simulink model "neural_network_and_real_data"  (Simulink 5.0)
settings: Solver=ode45  StartTime=0.0  StopTime=96  RelTol=1e-3
libraries: neural x7
settings Model: LastModifiedBy=Admin

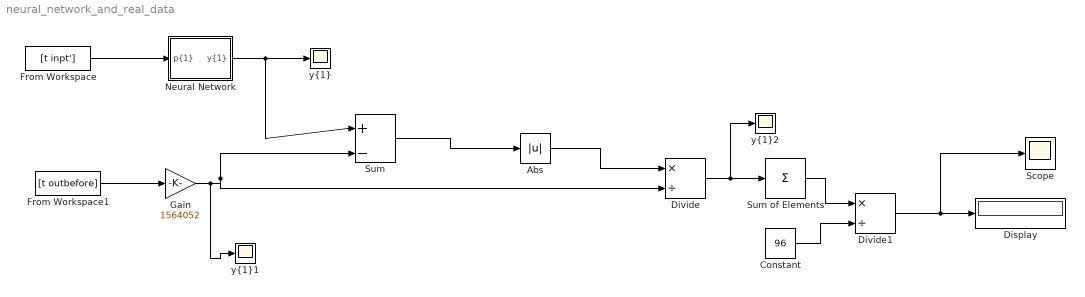
== system neural_network_and_real_data ==
  Abs : Abs  SaturateOnIntegerOverflow=on
  Constant : Constant  Value=96
  Display : Display
  Divide : Product  Inputs=*/  ShowAdditionalParam=on  OutDataTypeMode=double  OutScaling=2^-10
  Divide1 : Product  Inputs=*/  ShowAdditionalParam=on  OutDataTypeMode=double  OutScaling=2^-10
  From Workspace : FromWorkspace  VariableName=[t inpt']  SampleTime=0
  From Workspace1 : FromWorkspace  VariableName=[t outbefore]  SampleTime=0
  Gain : Gain  Gain=1564052  SaturateOnIntegerOverflow=on
  Neural Network : Subsystem
  Scope : Scope
  Sum : Sum  Inputs=|+-  SaturateOnIntegerOverflow=on
  Sum of Elements : Sum  Inputs=+  ShowAdditionalParam=on  OutDataTypeMode=double  OutScaling=2^-10
  "y{1}" : Scope
      settings: DataFormat=Array
  "y{1}1" : Scope
      settings: SaveName=ScopeData2  DataFormat=Array
  "y{1}2" : Scope
      settings: SaveName=ScopeData3  DataFormat=Array
  wires:
  From Workspace1/1 -> Gain/1
  Sum/1 -> Abs/1
  Abs/1 -> Divide/1
  Gain/1 -> Sum/2, Divide/2, "y{1}1"/1
  Divide/1 -> Sum of Elements/1, "y{1}2"/1
  Sum of Elements/1 -> Divide1/1
  Divide1/1 -> Display/1, Scope/1
  Constant/1 -> Divide1/2
  From Workspace/1 -> Neural Network/1("p{1}")
  Neural Network/1("y{1}") -> "y{1}"/1, Sum/1

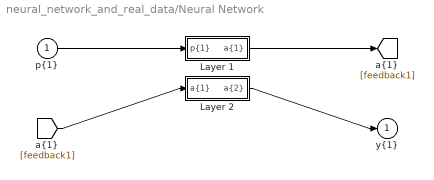
== system neural_network_and_real_data/Neural Network ==
  "p{1}" : Inport  PortDimensions=14  SampleTime=1
  Layer 1 : Subsystem
  Layer 2 : Subsystem
  "y{1}" : Outport  InitialOutput=0
  wires:
  "p{1}"/1 -> Layer 1/1("p{1}")
  Layer 1/1("a{1}") -> [feedback1]
  [feedback1] -> Layer 2/1("a{1} ")
  Layer 2/1("a{2}") -> "y{1}"/1

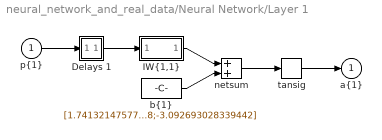
== system neural_network_and_real_data/Neural Network/Layer 1 ==
  "p{1}" : Inport  PortDimensions=14  SampleTime=1
  Delays 1 : Subsystem
      mask Display: disp('TDL')
  "IW{1,1}" : Subsystem
      mask Display: disp('weight')
  "b{1}" : Constant  Value=[1.7413214757740016;0.69735815383961486;-8.2527879365355368;-3.092693028339442]
      mask Display: disp('bias')
  netsum : Sum  Inputs=2  SaturateOnIntegerOverflow=on  InputSameDT=on
  tansig : neural/Transfer Functions/tansig
  "a{1}" : Outport  InitialOutput=[0;0;0;0]
  wires:
  "p{1}"/1 -> Delays 1/1("p{1}")
  Delays 1/1("pd{1,1}") -> "IW{1,1}"/1("pd{1,1}")
  "IW{1,1}"/1("iz{1,1}") -> netsum/1
  "b{1}"/1 -> netsum/2
  netsum/1 -> tansig/1
  tansig/1 -> "a{1}"/1

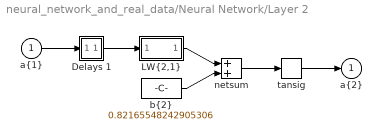
== system neural_network_and_real_data/Neural Network/Layer 2 ==
  "a{1} " : Inport  PortDimensions=4  SampleTime=1
  Delays 1 : Subsystem
      mask Display: disp('TDL')
  "LW{2,1}" : Subsystem
      mask Display: disp('weight')
  "b{2}" : Constant  Value=0.82165548242905306
      mask Display: disp('bias')
  netsum : Sum  Inputs=2  SaturateOnIntegerOverflow=on  InputSameDT=on
  tansig : neural/Transfer Functions/tansig
  "a{2}" : Outport  InitialOutput=0
  wires:
  "a{1} "/1 -> Delays 1/1("p{2}")
  Delays 1/1("pd{2,1}") -> "LW{2,1}"/1("ad{2,1}")
  "LW{2,1}"/1("lz{2,1}") -> netsum/1
  "b{2}"/1 -> netsum/2
  netsum/1 -> tansig/1
  tansig/1 -> "a{2}"/1

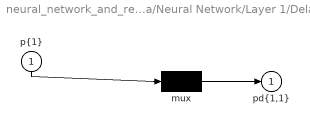
== system neural_network_and_real_data/Neural Network/Layer 1/Delays 1 ==
  "p{1}" : Inport  Orientation=down  PortDimensions=14  SampleTime=1
  mux : Mux  Inputs=1
  "pd{1,1}" : Outport
  wires:
  "p{1}"/1 -> mux/1
  mux/1 -> "pd{1,1}"/1

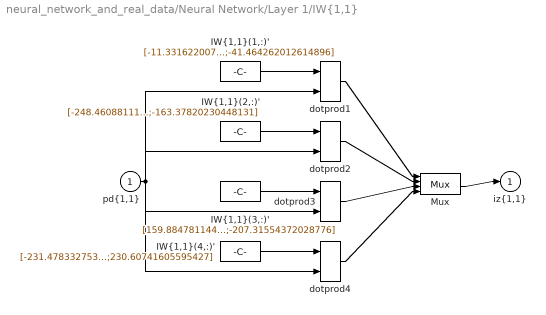
== system neural_network_and_real_data/Neural Network/Layer 1/IW{1,1} ==
  "pd{1,1}" : Inport  PortDimensions=14  SampleTime=1
  "IW{1,1}(1,:)'" : Constant  Value=[-11.331622007191116;480.76986123522266;-244.71826066692819;-215.36506776781869;117.68500710328458;961.37104772765292;-164.93584774087921;-123.71162401167672;-325.39584551772799;869.37046720143348;162.2602095339715;243.93099518166414;250.59760510926006;-41.464262012614896]
      mask Display: disp('weights')
  "IW{1,1}(2,:)'" : Constant  Value=[-248.46088111977173;592.96489870194205;-169.99826511296075;6.7210352268005842;-479.55640228789809;-945.29091142723746;-127.8654249967985;-4.8660732727339644;-66.740410653909109;-1194.9112669366377;-592.82533601042496;-973.13653211376027;-59.240012956465101;-163.37820230448131]
      mask Display: disp('weights')
  "IW{1,1}(3,:)'" : Constant  Value=[159.88478114481589;510.1389358159833;-666.21169528304029;122.42329706388527;73.862813450675262;1057.5895380083077;83.172587324821478;-83.831737188744668;-130.97395062127208;-1449.259370525705;-445.13943115786509;-243.29810900368994;-218.09638607845807;-207.31554372028776]
      mask Display: disp('weights')
  "IW{1,1}(4,:)'" : Constant  Value=[-231.47833275364465;432.94058782940772;481.12543704920199;-189.06868666119615;108.88512919705389;634.60855022269948;33.238156784438438;-420.44459886676248;-87.906302700763874;457.34879761095931;-361.47211045958676;296.27717948861425;-94.358408155950343;230.60741605595427]
      mask Display: disp('weights')
  Mux : Mux
  dotprod{1..4} (4 alike) : neural/Weight Functions/dotprod
  "iz{1,1}" : Outport
  wires:
  "IW{1,1}(1,:)'"/1 -> dotprod1/1
  "pd{1,1}"/1 -> dotprod1/2, dotprod2/2, dotprod3/2, dotprod4/2
  dotprod1/1 -> Mux/1
  "IW{1,1}(2,:)'"/1 -> dotprod2/1
  dotprod2/1 -> Mux/2
  "IW{1,1}(3,:)'"/1 -> dotprod3/1
  dotprod3/1 -> Mux/3
  "IW{1,1}(4,:)'"/1 -> dotprod4/1
  dotprod4/1 -> Mux/4
  Mux/1 -> "iz{1,1}"/1

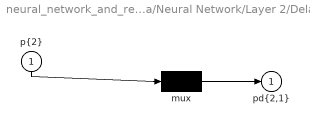
== system neural_network_and_real_data/Neural Network/Layer 2/Delays 1 ==
  "p{2}" : Inport  Orientation=down  PortDimensions=4  SampleTime=1
  mux : Mux  Inputs=1
  "pd{2,1}" : Outport
  wires:
  "p{2}"/1 -> mux/1
  mux/1 -> "pd{2,1}"/1

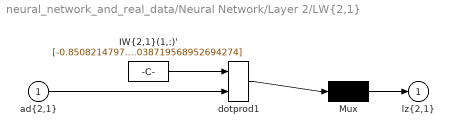
== system neural_network_and_real_data/Neural Network/Layer 2/LW{2,1} ==
  "ad{2,1}" : Inport  PortDimensions=4  SampleTime=1
  "IW{2,1}(1,:)'" : Constant  Value=[-0.85082147972736011;-0.0020020092638200438;0.0014643763862159755;-0.038719568952694274]
      mask Display: disp('weights')
  Mux : Mux  Inputs=1
  dotprod1 : neural/Weight Functions/dotprod
  "lz{2,1}" : Outport
  wires:
  "IW{2,1}(1,:)'"/1 -> dotprod1/1
  "ad{2,1}"/1 -> dotprod1/2
  dotprod1/1 -> Mux/1
  Mux/1 -> "lz{2,1}"/1
